simulink model "impulse_ex_2"  (R2024a)
settings: Solver=VariableStepAuto  StartTime=0.0  StopTime=6.23456  RelTol=1e-3
undefined symbols (not defined in the file or in its folder): sys
libraries: simulink x1
settings Model: Creator=grouleau  LastModifiedBy=grouleau

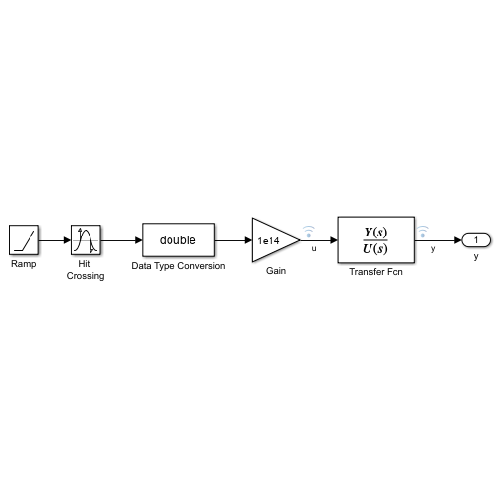
[thumbnail: Simulink's stored preview of the top-level diagram]
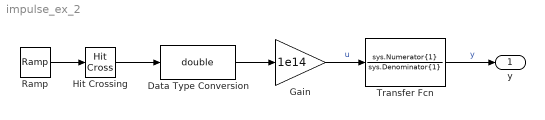
== system impulse_ex_2 ==
  Data Type Conversion : DataTypeConversion  OutDataTypeStr=double  SaturateOnIntegerOverflow=off  RndMeth=Floor
  Gain : Gain  Gain=1e14
  Hit Crossing : HitCross  HitCrossingOffset=1.23456
  Ramp : simulink/Sources/Ramp  slope=1  start=0  InitialOutput=0
  Transfer Fcn : TransferFcn  Numerator=sys.Numerator{1}  Denominator=sys.Denominator{1}
  y : Outport
  wires:
  Transfer Fcn/1 -> y/1  "y"
  Ramp/1 -> Hit Crossing/1
  Hit Crossing/1 -> Data Type Conversion/1
  Data Type Conversion/1 -> Gain/1
  Gain/1 -> Transfer Fcn/1  "u"
